simulink model "prob_1"  (R2020b)
settings: Solver=VariableStepAuto  StartTime=0.0  StopTime=10.0  RelTol=1e-3
model workspace (MAT data in the model file):
  K1 = 50
  K12 = 0
  M1 = 1000
  M2 = 0
  b = 50
settings Model: Creator=Lakshmi  LastModifiedBy=Lakshmi

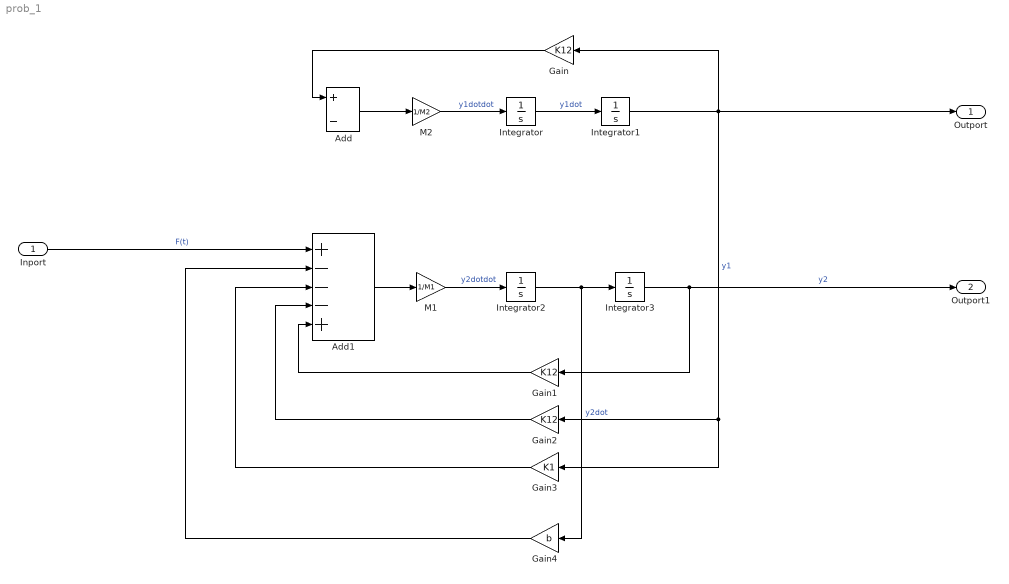
== system prob_1 ==
  Inport : Inport
  Add : Sum  Inputs=+-
  Add1 : Sum  Inputs=+---+
  Gain : Gain  Gain=K12
  Gain1 : Gain  Gain=K12
  Gain2 : Gain  Gain=K12
  Gain3 : Gain  Gain=K1
  Gain4 : Gain  Gain=b
  Integrator{,1..3} (4 alike) : Integrator
  M1 : Gain  Gain=1/M1
  M2 : Gain  Gain=1/M2
  Outport : Outport
  Outport1 : Outport  Port=2
  wires:
  Add/1 -> M2/1
  M2/1 -> Integrator/1  "y1dotdot"
  Integrator/1 -> Integrator1/1  "y1dot"
  Integrator1/1 -> Gain3/1, Gain2/1, Gain/1, Outport/1  "y1"
  Gain/1 -> Add/1
  Inport/1 -> Add1/1  "F(t)"
  Add1/1 -> M1/1
  M1/1 -> Integrator2/1  "y2dotdot"
  Integrator2/1 -> Gain4/1, Integrator3/1  "y2dot"
  Integrator3/1 -> Gain1/1, Outport1/1  "y2"
  Gain1/1 -> Add1/5
  Gain2/1 -> Add1/4
  Gain3/1 -> Add1/3
  Gain4/1 -> Add1/2
